simulink model "substation_exp11"  (R2021b)
settings: Solver=VariableStepAuto  StartTime=0.0  StopTime=10  RelTol=1e-3
undefined symbols (not defined in the file): a
libraries: spsThreePhaseBreakerLib x13, spsThreePhaseVIMeasurementLib x10, spsRMSLib x4, spsThreePhaseSeriesRLCLoadLib x4, spsThreePhaseSourceLib x3, spsThreePhaseTransformerTwoWindingsLib x3, spsThreePhaseFaultLib x1, spspowerguiLib x1
settings Model: Creator=SAI KUMAR  LastModifiedBy=SAI KUMAR
settings SolverCC: ZeroCrossAlgorithm=Adaptive
settings DebuggingCC: IgnoredZcDiagnostic=none

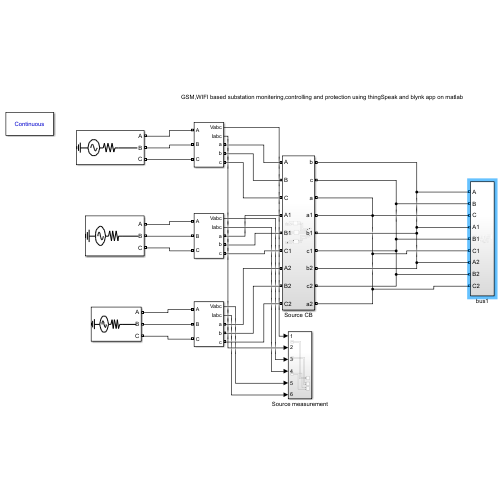
[thumbnail: Simulink's stored preview of the top-level diagram]
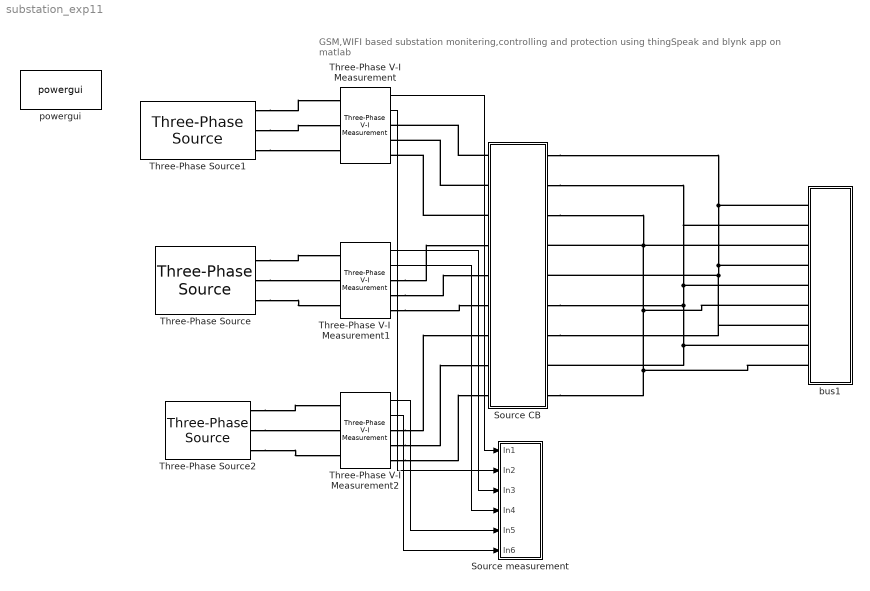
== system substation_exp11 ==
  note: GSM,WIFI based substation monitering,controlling and protection using thingSpeak and blynk app on matlab
  Source CB : Subsystem
  Source measurement : Subsystem
  Three-Phase V-I Measurement : spsThreePhaseVIMeasurementLib/Three-Phase V-I Measurement  VoltageMeasurement=phase-to-ground  SetLabelV=off  LabelV=Vabc  Vpu=off  VpuLL=off  CurrentMeasurement=yes  SetLabelI=off  LabelI=Iabc  Ipu=off  Pbase=100e6  Vbase=500e3  OutputType=Complex  PhasorSimulation=off  PSBequivalent=0
  Three-Phase V-I Measurement1 : spsThreePhaseVIMeasurementLib/Three-Phase V-I Measurement  VoltageMeasurement=phase-to-ground  SetLabelV=off  LabelV=Vabc  Vpu=off  VpuLL=off  CurrentMeasurement=yes  SetLabelI=off  LabelI=Iabc  Ipu=off  Pbase=100e6  Vbase=500e3  OutputType=Complex  PhasorSimulation=off  PSBequivalent=0
  Three-Phase V-I Measurement2 : spsThreePhaseVIMeasurementLib/Three-Phase V-I Measurement  VoltageMeasurement=phase-to-ground  SetLabelV=off  LabelV=Vabc  Vpu=off  VpuLL=off  CurrentMeasurement=yes  SetLabelI=off  LabelI=Iabc  Ipu=off  Pbase=100e6  Vbase=500e3  OutputType=Complex  PhasorSimulation=off  PSBequivalent=0
  Three-Phase Source : spsThreePhaseSourceLib/Three-Phase Source  InternalConnection=Yg  VoltagePhases=off  Voltage=11000  PhaseAngle=0  Voltage_phases=[25e3 25e3 25e3]/sqrt(3)  PhaseAngles_phases=[0 -120 +120]  Frequency=50  NonIdealSource=on  SpecifyImpedance=off  Resistance=0.8929  Inductance=0  ShortCircuitLevel=100e6  BaseVoltage=11000  XRratio=7  BusType=swing  Pref=10e3  Qref=0  Prefabc=[10e3, 10e3, 10e3]  Qrefabc=[0, 0, 0]  Qmin=-inf  Qmax=inf
  Three-Phase Source1 : spsThreePhaseSourceLib/Three-Phase Source  InternalConnection=Yg  VoltagePhases=off  Voltage=11000  PhaseAngle=0  Voltage_phases=[25e3 25e3 25e3]/sqrt(3)  PhaseAngles_phases=[0 -120 +120]  Frequency=50  NonIdealSource=on  SpecifyImpedance=off  Resistance=0.8929  Inductance=0  ShortCircuitLevel=100e6  BaseVoltage=11000  XRratio=7  BusType=swing  Pref=10e3  Qref=0  Prefabc=[10e3, 10e3, 10e3]  Qrefabc=[0, 0, 0]  Qmin=-inf  Qmax=inf
  Three-Phase Source2 : spsThreePhaseSourceLib/Three-Phase Source  InternalConnection=Yg  VoltagePhases=off  Voltage=11000  PhaseAngle=0  Voltage_phases=[25e3 25e3 25e3]/sqrt(3)  PhaseAngles_phases=[0 -120 +120]  Frequency=50  NonIdealSource=on  SpecifyImpedance=off  Resistance=0.8929  Inductance=0  ShortCircuitLevel=100e6  BaseVoltage=11000  XRratio=7  BusType=swing  Pref=10e3  Qref=0  Prefabc=[10e3, 10e3, 10e3]  Qrefabc=[0, 0, 0]  Qmin=-inf  Qmax=inf
  bus1 : Subsystem
  powergui : spspowerguiLib/powergui  Priority=1  SimulationMode=Continuous  SampleTime=50e-6  frequency=60  Iterations=50  frequencyindice=50  Pbase=100e6  ErrMax=1e-4  UnitsV=kV  UnitsW=MW  buscounter=0  FunctionMessages=off  echomessages=off  EnableUseOfTLC=off  CurrentSourceSwitches=off  DisableSnubberDevices=off  DisableRonSwitches=off  DisableVfSwitches=off  DisplayEquations=off  AutomaticDiscreteSolvers=off  SolverType=Tustin/Backward Euler (TBE)  Interpol=off  ExternalGateDelay=off  methode=off  Ts=100  x0status=blocks  SPID=on  SwTol=0  HookPort=off  NonlinearTolerance=1e-4  nMaxIteration=100  ContinueOnMaxIteration=off  RestoreLinks=warning  ResistiveCurrentMeasurement=off  Frange=[0:2:500]  Ylog=off  Xlog=on  ShowGrid=off  save=off  variable=ZData  structure=0  ZoomFFT=off  StartTime=0.0  cycles=1  DisplayStyle=1  fundamental=60  FreqAxis=off  MaxFrequency=1000  frequencyindicesteady=1  RmsSteady=1  display=off
  wires:
  Three-Phase V-I Measurement/1 -> Source measurement/1(In1)
  Three-Phase V-I Measurement/2 -> Source measurement/2(In2)
  Three-Phase V-I Measurement1/1 -> Source measurement/3(In3)
  Three-Phase V-I Measurement1/2 -> Source measurement/4(In4)
  Three-Phase V-I Measurement2/1 -> Source measurement/5(In5)
  Three-Phase V-I Measurement2/2 -> Source measurement/6(In6)
  connections:
  bus1/LConn1 -- Source CB/RConn5 -- Source CB/RConn7 -- bus1/LConn7 -- bus1/LConn4 -- Source CB/RConn1
  Three-Phase Source2/RConn1 -- Three-Phase V-I Measurement2/LConn1
  Three-Phase Source2/RConn2 -- Three-Phase V-I Measurement2/LConn2
  Three-Phase Source2/RConn3 -- Three-Phase V-I Measurement2/LConn3
  Three-Phase Source/RConn1 -- Three-Phase V-I Measurement1/LConn1
  Three-Phase Source/RConn2 -- Three-Phase V-I Measurement1/LConn2
  Three-Phase Source/RConn3 -- Three-Phase V-I Measurement1/LConn3
  Three-Phase Source1/RConn1 -- Three-Phase V-I Measurement/LConn1
  Three-Phase Source1/RConn2 -- Three-Phase V-I Measurement/LConn2
  Three-Phase Source1/RConn3 -- Three-Phase V-I Measurement/LConn3
  bus1/LConn9 -- Source CB/RConn9 -- bus1/LConn6 -- bus1/LConn3 -- Source CB/RConn3 -- Source CB/RConn4
  bus1/LConn5 -- Source CB/RConn2 -- bus1/LConn2 -- Source CB/RConn6 -- Source CB/RConn8 -- bus1/LConn8
  Source CB/LConn1 -- Three-Phase V-I Measurement/RConn1
  Source CB/LConn2 -- Three-Phase V-I Measurement/RConn2
  Source CB/LConn3 -- Three-Phase V-I Measurement/RConn3
  Three-Phase V-I Measurement1/RConn1 -- Source CB/LConn4
  Three-Phase V-I Measurement1/RConn2 -- Source CB/LConn5
  Three-Phase V-I Measurement1/RConn3 -- Source CB/LConn6
  Three-Phase V-I Measurement2/RConn1 -- Source CB/LConn7
  Three-Phase V-I Measurement2/RConn2 -- Source CB/LConn8
  Three-Phase V-I Measurement2/RConn3 -- Source CB/LConn9

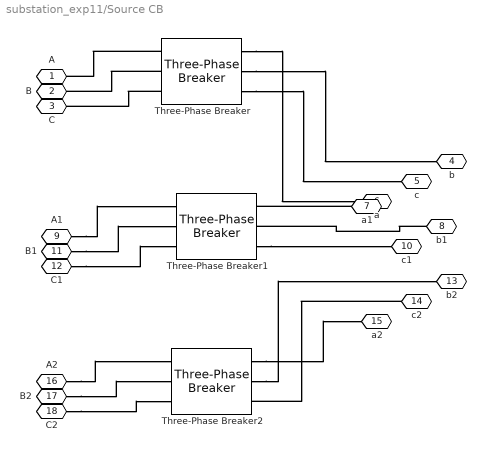
== system substation_exp11/Source CB ==
  Three-Phase Breaker : spsThreePhaseBreakerLib/Three-Phase Breaker  InitialState=closed  SwitchA=on  SwitchB=on  SwitchC=on  SwitchTimes="[1/60  5/60]"  External=off  BreakerResistance=0.01  SnubberResistance=1e6  SnubberCapacitance=inf  Measurements=None
  Three-Phase Breaker1 : spsThreePhaseBreakerLib/Three-Phase Breaker  InitialState=closed  SwitchA=on  SwitchB=on  SwitchC=on  SwitchTimes="[1/60  5/60]"  External=off  BreakerResistance=0.01  SnubberResistance=1e6  SnubberCapacitance=inf  Measurements=None
  Three-Phase Breaker2 : spsThreePhaseBreakerLib/Three-Phase Breaker  InitialState=closed  SwitchA=on  SwitchB=on  SwitchC=on  SwitchTimes="[1/60  5/60]"  External=off  BreakerResistance=0.01  SnubberResistance=1e6  SnubberCapacitance=inf  Measurements=None
  A : PMIOPort  Side=Left
  B : PMIOPort  Port=2  Side=Left
  C : PMIOPort  Port=3  Side=Left
  b : PMIOPort  Port=4  Side=Right
  c : PMIOPort  Port=5  Side=Right
  a : PMIOPort  Port=6  Side=Right
  a1 : PMIOPort  Port=7  Side=Right
  b1 : PMIOPort  Port=8  Side=Right
  A1 : PMIOPort  Port=9  Side=Left
  c1 : PMIOPort  Port=10  Side=Right
  B1 : PMIOPort  Port=11  Side=Left
  C1 : PMIOPort  Port=12  Side=Left
  b2 : PMIOPort  Port=13  Side=Right
  c2 : PMIOPort  Port=14  Side=Right
  a2 : PMIOPort  Port=15  Side=Right
  A2 : PMIOPort  Port=16  Side=Left
  B2 : PMIOPort  Port=17  Side=Left
  C2 : PMIOPort  Port=18  Side=Left
  connections:
  Three-Phase Breaker2/RConn1 -- a2/RConn1
  Three-Phase Breaker2/RConn2 -- b2/RConn1
  A1/RConn1 -- Three-Phase Breaker1/LConn1
  B1/RConn1 -- Three-Phase Breaker1/LConn2
  b1/RConn1 -- Three-Phase Breaker1/RConn2
  C2/RConn1 -- Three-Phase Breaker2/LConn3
  Three-Phase Breaker/RConn1 -- a/RConn1
  c2/RConn1 -- Three-Phase Breaker2/RConn3
  Three-Phase Breaker/RConn3 -- c/RConn1
  Three-Phase Breaker/LConn1 -- A/RConn1
  a1/RConn1 -- Three-Phase Breaker1/RConn1
  B2/RConn1 -- Three-Phase Breaker2/LConn2
  C1/RConn1 -- Three-Phase Breaker1/LConn3
  Three-Phase Breaker/LConn2 -- B/RConn1
  Three-Phase Breaker1/RConn3 -- c1/RConn1
  A2/RConn1 -- Three-Phase Breaker2/LConn1
  Three-Phase Breaker/RConn2 -- b/RConn1
  Three-Phase Breaker/LConn3 -- C/RConn1

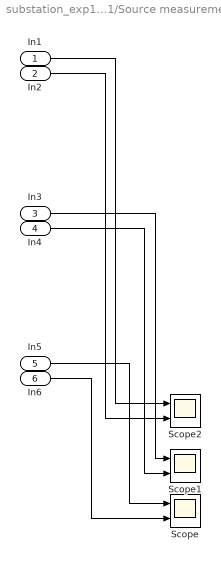
== system substation_exp11/Source measurement ==
  In1 : Inport
  In2 : Inport  Port=2
  In3 : Inport  Port=3
  In4 : Inport  Port=4
  In5 : Inport  Port=5
  In6 : Inport  Port=6
  Scope : Scope  NumInputPorts=2
  Scope1 : Scope  NumInputPorts=2
  Scope2 : Scope  NumInputPorts=2
  wires:
  In5/1 -> Scope/1
  In6/1 -> Scope/2
  In2/1 -> Scope2/2
  In4/1 -> Scope1/2
  In3/1 -> Scope1/1
  In1/1 -> Scope2/1

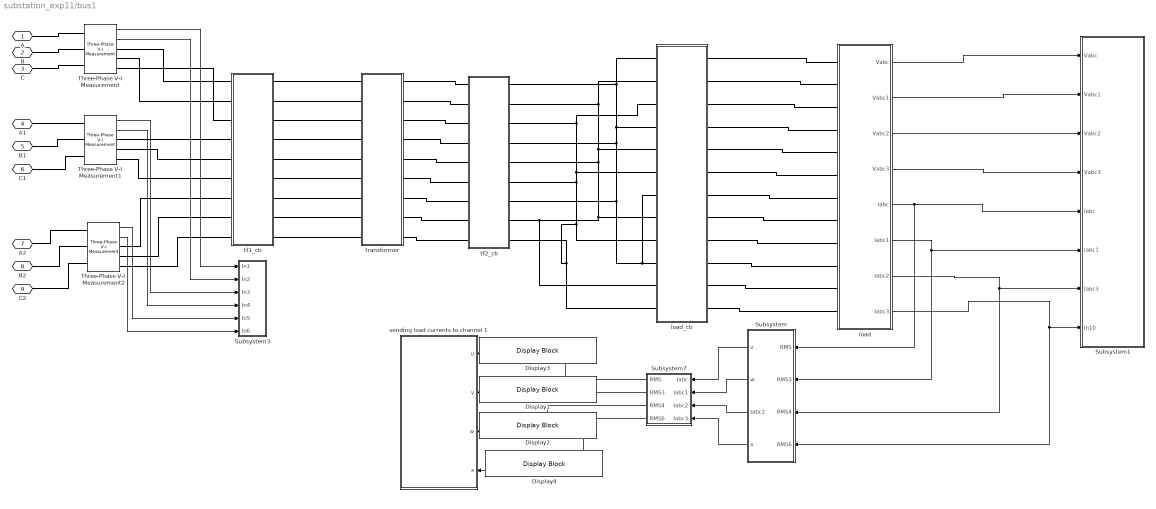
== system substation_exp11/bus1 ==
  Display{1..4} (4 alike) : DisplayBlock  LabelPosition=Hide  Format=short  Transparency=1
  Subsystem : Subsystem
  Subsystem1 : Subsystem
  Subsystem3 : Subsystem
  Subsystem7 : Subsystem
  Three-Phase V-I Measurement : spsThreePhaseVIMeasurementLib/Three-Phase V-I Measurement  VoltageMeasurement=phase-to-ground  SetLabelV=off  LabelV=Vabc  Vpu=off  VpuLL=off  CurrentMeasurement=yes  SetLabelI=off  LabelI=Iabc  Ipu=off  Pbase=100e6  Vbase=500e3  OutputType=Complex  PhasorSimulation=off  PSBequivalent=0
  Three-Phase V-I Measurement1 : spsThreePhaseVIMeasurementLib/Three-Phase V-I Measurement  VoltageMeasurement=phase-to-ground  SetLabelV=off  LabelV=Vabc  Vpu=off  VpuLL=off  CurrentMeasurement=yes  SetLabelI=off  LabelI=Iabc  Ipu=off  Pbase=100e6  Vbase=500e3  OutputType=Complex  PhasorSimulation=off  PSBequivalent=0
  Three-Phase V-I Measurement2 : spsThreePhaseVIMeasurementLib/Three-Phase V-I Measurement  VoltageMeasurement=phase-to-ground  SetLabelV=off  LabelV=Vabc  Vpu=off  VpuLL=off  CurrentMeasurement=yes  SetLabelI=off  LabelI=Iabc  Ipu=off  Pbase=100e6  Vbase=500e3  OutputType=Complex  PhasorSimulation=off  PSBequivalent=0
  load : Subsystem
  load_cb : Subsystem
  sending load currents to channel 1 : MATLAB Function  TreatAsAtomicUnit=on
  tf1_cb : Subsystem
  tf2_cb : Subsystem
  transformer : Subsystem
  A : PMIOPort  Side=Left
  B : PMIOPort  Port=2  Side=Left
  C : PMIOPort  Port=3  Side=Left
  A1 : PMIOPort  Port=4  Side=Left
  B1 : PMIOPort  Port=5  Side=Left
  C1 : PMIOPort  Port=6  Side=Left
  A2 : PMIOPort  Port=7  Side=Left
  B2 : PMIOPort  Port=8  Side=Left
  C2 : PMIOPort  Port=9  Side=Left
  wires:
  Three-Phase V-I Measurement/1 -> Subsystem3/1(In1)
  Three-Phase V-I Measurement/2 -> Subsystem3/2(In2)
  Three-Phase V-I Measurement1/1 -> Subsystem3/3(In3)
  Three-Phase V-I Measurement1/2 -> Subsystem3/4(In4)
  Three-Phase V-I Measurement2/1 -> Subsystem3/5(In5)
  Three-Phase V-I Measurement2/2 -> Subsystem3/6(In6)
  load/6(Iabc1) -> Subsystem1/6(Iabc1), Subsystem/2(RMS3)
  load/8(Iabc3) -> Subsystem/4(RMS6), Subsystem1/8(In10)
  load/1(Vabc) -> Subsystem1/1(Vabc)
  load/2(Vabc1) -> Subsystem1/2(Vabc1)
  load/3(Vabc2) -> Subsystem1/3(Vabc2)
  load/4(Vabc3) -> Subsystem1/4(Vabc3)
  load/5(Iabc) -> Subsystem/1(RMS), Subsystem1/5(Iabc)
  load/7(Iabc2) -> Subsystem/3(RMS4), Subsystem1/7(Iabc3)
  Subsystem/1(v) -> Subsystem7/1(Iabc)
  Subsystem/2(w) -> Subsystem7/2(Iabc1)
  Subsystem/3(Iabc2) -> Subsystem7/3(Iabc2)
  Subsystem/4(x) -> Subsystem7/4(Iabc3)
  Subsystem7/1(RMS) -> sending load currents to channel 1/1(u)
  Subsystem7/2(RMS3) -> sending load currents to channel 1/2(v)
  Subsystem7/3(RMS4) -> sending load currents to channel 1/3(w)
  Subsystem7/4(RMS6) -> sending load currents to channel 1/4(x)
  connections:
  Three-Phase V-I Measurement/LConn1 -- A/RConn1
  Three-Phase V-I Measurement/LConn2 -- B/RConn1
  Three-Phase V-I Measurement/LConn3 -- C/RConn1
  Three-Phase V-I Measurement1/LConn1 -- A1/RConn1
  Three-Phase V-I Measurement1/LConn2 -- B1/RConn1
  Three-Phase V-I Measurement1/LConn3 -- C1/RConn1
  Three-Phase V-I Measurement2/LConn1 -- A2/RConn1
  Three-Phase V-I Measurement2/LConn2 -- B2/RConn1
  Three-Phase V-I Measurement2/LConn3 -- C2/RConn1
  Three-Phase V-I Measurement/RConn1 -- tf1_cb/LConn1
  Three-Phase V-I Measurement/RConn2 -- tf1_cb/LConn2
  Three-Phase V-I Measurement/RConn3 -- tf1_cb/LConn3
  Three-Phase V-I Measurement1/RConn1 -- tf1_cb/LConn4
  Three-Phase V-I Measurement1/RConn2 -- tf1_cb/LConn5
  Three-Phase V-I Measurement1/RConn3 -- tf1_cb/LConn6
  Three-Phase V-I Measurement2/RConn1 -- tf1_cb/LConn7
  Three-Phase V-I Measurement2/RConn2 -- tf1_cb/LConn8
  Three-Phase V-I Measurement2/RConn3 -- tf1_cb/LConn9
  tf2_cb/RConn1 -- tf2_cb/RConn7 -- load_cb/LConn10 -- load_cb/LConn7 -- tf2_cb/RConn4 -- load_cb/LConn4 -- load_cb/LConn1
  tf2_cb/RConn2 -- load_cb/LConn11 -- tf2_cb/RConn8 -- load_cb/LConn8 -- tf2_cb/RConn5 -- load_cb/LConn5 -- load_cb/LConn2
  tf2_cb/RConn3 -- load_cb/LConn12 -- tf2_cb/RConn9 -- load_cb/LConn9 -- tf2_cb/RConn6 -- load_cb/LConn6 -- load_cb/LConn3
  load/LConn1 -- load_cb/RConn1
  load/LConn2 -- load_cb/RConn2
  load_cb/RConn3 -- load/LConn3
  load_cb/RConn4 -- load/LConn4
  load_cb/RConn5 -- load/LConn5
  load_cb/RConn6 -- load/LConn6
  load/LConn7 -- load_cb/RConn7
  load_cb/RConn8 -- load/LConn8
  load_cb/RConn9 -- load/LConn9
  load_cb/RConn10 -- load/LConn10
  load_cb/RConn11 -- load/LConn11
  load_cb/RConn12 -- load/LConn12
  transformer/LConn1 -- tf1_cb/RConn1
  transformer/LConn2 -- tf1_cb/RConn2
  tf2_cb/LConn1 -- transformer/RConn1
  transformer/LConn3 -- tf1_cb/RConn3
  tf2_cb/LConn2 -- transformer/RConn2
  transformer/LConn4 -- tf1_cb/RConn4
  tf2_cb/LConn3 -- transformer/RConn3
  transformer/LConn5 -- tf1_cb/RConn5
  tf2_cb/LConn4 -- transformer/RConn4
  transformer/LConn6 -- tf1_cb/RConn6
  tf2_cb/LConn5 -- transformer/RConn5
  transformer/LConn7 -- tf1_cb/RConn7
  tf2_cb/LConn6 -- transformer/RConn6
  transformer/LConn8 -- tf1_cb/RConn8
  tf2_cb/LConn7 -- transformer/RConn7
  transformer/LConn9 -- tf1_cb/RConn9
  tf2_cb/LConn8 -- transformer/RConn8
  tf2_cb/LConn9 -- transformer/RConn9

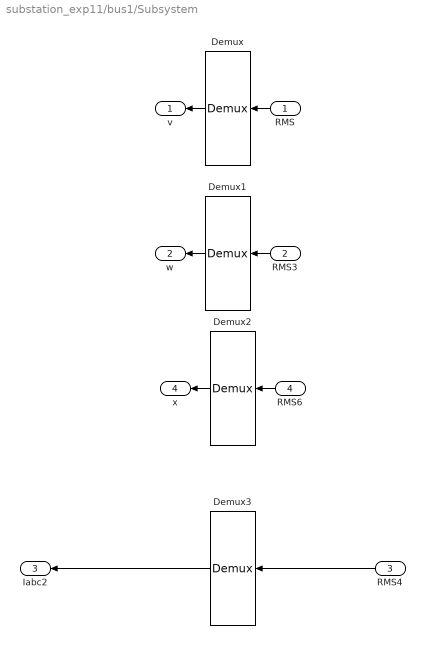
== system substation_exp11/bus1/Subsystem ==
  RMS : Inport
  RMS3 : Inport  Port=2
  RMS4 : Inport  Port=3
  RMS6 : Inport  Port=4
  Demux{,1..3} (4 alike) : Demux  Outputs=3
  v : Outport
  w : Outport  Port=2
  Iabc2 : Outport  Port=3
  x : Outport  Port=4
  wires:
  RMS3/1 -> Demux1/1
  Demux3/2 -> Iabc2/1
  RMS4/1 -> Demux3/1
  Demux1/2 -> w/1
  Demux2/2 -> x/1
  RMS/1 -> Demux/1
  RMS6/1 -> Demux2/1
  Demux/2 -> v/1

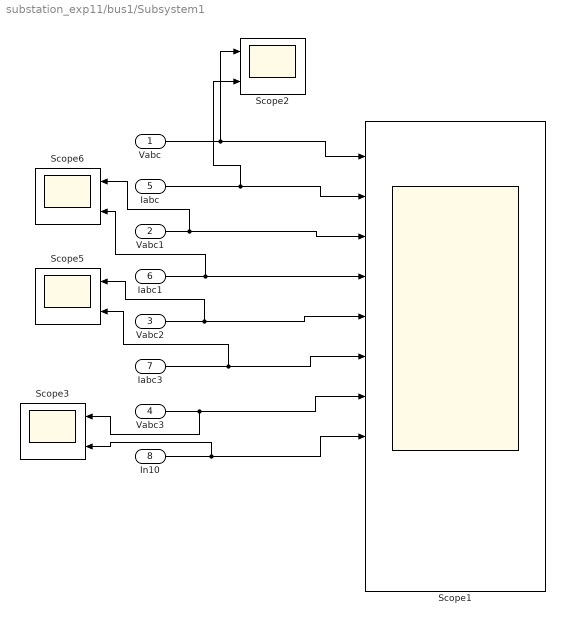
== system substation_exp11/bus1/Subsystem1 ==
  Vabc : Inport
  Vabc1 : Inport  Port=2
  Vabc2 : Inport  Port=3
  Vabc3 : Inport  Port=4
  Iabc : Inport  Port=5
  Iabc1 : Inport  Port=6
  Iabc3 : Inport  Port=7
  In10 : Inport  Port=8
  Scope1 : Scope  NumInputPorts=11
  Scope{2..3,5..6} (4 alike) : Scope  NumInputPorts=2
  wires:
  Iabc3/1 -> Scope5/2, Scope1/6
  Iabc1/1 -> Scope1/4, Scope6/2
  Vabc3/1 -> Scope3/1, Scope1/7
  Vabc2/1 -> Scope5/1, Scope1/5
  Vabc/1 -> Scope2/1, Scope1/1
  Iabc/1 -> Scope2/2, Scope1/2
  Vabc1/1 -> Scope1/3, Scope6/1
  In10/1 -> Scope3/2, Scope1/8

== system substation_exp11/bus1/Subsystem3 ==
  In1 : Inport
  In2 : Inport  Port=2
  In3 : Inport  Port=3
  In4 : Inport  Port=4
  In5 : Inport  Port=5
  In6 : Inport  Port=6
  Scope : Scope  NumInputPorts=2
  Scope3 : Scope  NumInputPorts=2
  Scope4 : Scope  NumInputPorts=2
  wires:
  In4/1 -> Scope3/2
  In1/1 -> Scope/1
  In3/1 -> Scope3/1
  In2/1 -> Scope/2
  In6/1 -> Scope4/2
  In5/1 -> Scope4/1

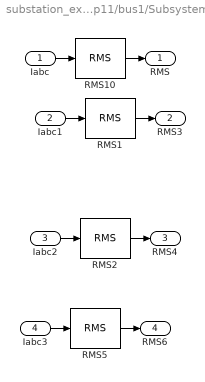
== system substation_exp11/bus1/Subsystem7 ==
  Iabc : Inport
  Iabc1 : Inport  Port=2
  Iabc2 : Inport  Port=3
  Iabc3 : Inport  Port=4
  RMS{1..2,5,10} (4 alike) : spsRMSLib/RMS  TrueRMS=on  Freq=50  RMSInit=0  Ts=a
  RMS : Outport
  RMS3 : Outport  Port=2
  RMS4 : Outport  Port=3
  RMS6 : Outport  Port=4
  wires:
  Iabc1/1 -> RMS1/1
  Iabc2/1 -> RMS2/1
  Iabc3/1 -> RMS5/1
  RMS5/1 -> RMS6/1
  Iabc/1 -> RMS10/1
  RMS2/1 -> RMS4/1
  RMS1/1 -> RMS3/1
  RMS10/1 -> RMS/1

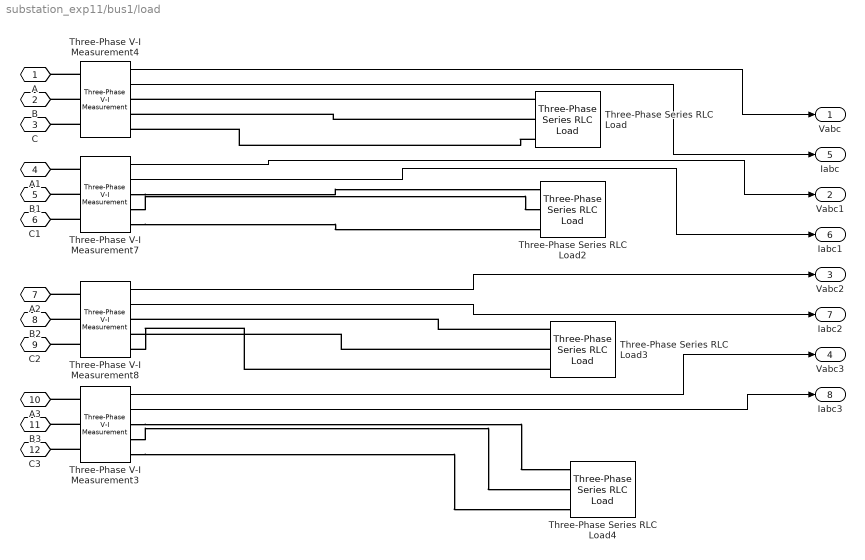
== system substation_exp11/bus1/load ==
  Three-Phase Series RLC Load : spsThreePhaseSeriesRLCLoadLib/Three-Phase Series RLC Load  LConnTagsString=A|B|C  Configuration=Y (grounded)  NominalVoltage=415  Vabc=[1e3 1e3 1e3]  Vabcp=[1e3 1e3 1e3]  NominalFrequency=50  UnbalancedPower=off  ActivePower=1000  InductivePower=0  CapacitivePower=0  Pabc=[10e3 9e3 11e3]  QLabc=[100 90 110]  QCabc=[100 90 110]  Pabcp=[10e3 9e3 11e3]  QLabcp=[100 90 110]  QCabcp=[100 90 110]  Measurements=None  LoadType=constant Z
  Three-Phase Series RLC Load2 : spsThreePhaseSeriesRLCLoadLib/Three-Phase Series RLC Load  LConnTagsString=A|B|C  Configuration=Y (grounded)  NominalVoltage=415  Vabc=[1e3 1e3 1e3]  Vabcp=[1e3 1e3 1e3]  NominalFrequency=50  UnbalancedPower=off  ActivePower=10e3  InductivePower=0  CapacitivePower=0  Pabc=[10e3 9e3 11e3]  QLabc=[100 90 110]  QCabc=[100 90 110]  Pabcp=[10e3 9e3 11e3]  QLabcp=[100 90 110]  QCabcp=[100 90 110]  Measurements=None  LoadType=constant Z
  Three-Phase Series RLC Load3 : spsThreePhaseSeriesRLCLoadLib/Three-Phase Series RLC Load  LConnTagsString=A|B|C  Configuration=Y (grounded)  NominalVoltage=415  Vabc=[1e3 1e3 1e3]  Vabcp=[1e3 1e3 1e3]  NominalFrequency=50  UnbalancedPower=off  ActivePower=10e3  InductivePower=0  CapacitivePower=0  Pabc=[10e3 9e3 11e3]  QLabc=[100 90 110]  QCabc=[100 90 110]  Pabcp=[10e3 9e3 11e3]  QLabcp=[100 90 110]  QCabcp=[100 90 110]  Measurements=None  LoadType=constant Z
  Three-Phase Series RLC Load4 : spsThreePhaseSeriesRLCLoadLib/Three-Phase Series RLC Load  LConnTagsString=A|B|C  Configuration=Y (grounded)  NominalVoltage=415  Vabc=[1e3 1e3 1e3]  Vabcp=[1e3 1e3 1e3]  NominalFrequency=50  UnbalancedPower=off  ActivePower=10e6  InductivePower=0  CapacitivePower=0  Pabc=[10e3 9e3 11e3]  QLabc=[100 90 110]  QCabc=[100 90 110]  Pabcp=[10e3 9e3 11e3]  QLabcp=[100 90 110]  QCabcp=[100 90 110]  Measurements=None  LoadType=constant Z
  Three-Phase V-I Measurement{3..4,7..8} (4 alike) : spsThreePhaseVIMeasurementLib/Three-Phase V-I Measurement  VoltageMeasurement=phase-to-phase  SetLabelV=off  LabelV=Vabc  Vpu=off  VpuLL=off  CurrentMeasurement=yes  SetLabelI=off  LabelI=Iabc  Ipu=off  Pbase=100e6  Vbase=500e3  OutputType=Complex  PhasorSimulation=off  PSBequivalent=0
  A : PMIOPort  Side=Left
  B : PMIOPort  Port=2  Side=Left
  C : PMIOPort  Port=3  Side=Left
  A1 : PMIOPort  Port=4  Side=Left
  B1 : PMIOPort  Port=5  Side=Left
  C1 : PMIOPort  Port=6  Side=Left
  A2 : PMIOPort  Port=7  Side=Left
  B2 : PMIOPort  Port=8  Side=Left
  C2 : PMIOPort  Port=9  Side=Left
  A3 : PMIOPort  Port=10  Side=Left
  B3 : PMIOPort  Port=11  Side=Left
  C3 : PMIOPort  Port=12  Side=Left
  Vabc : Outport
  Vabc1 : Outport  Port=2
  Vabc2 : Outport  Port=3
  Vabc3 : Outport  Port=4
  Iabc : Outport  Port=5
  Iabc1 : Outport  Port=6
  Iabc2 : Outport  Port=7
  Iabc3 : Outport  Port=8
  wires:
  Three-Phase V-I Measurement7/2 -> Iabc1/1
  Three-Phase V-I Measurement4/2 -> Iabc/1
  Three-Phase V-I Measurement8/2 -> Iabc2/1
  Three-Phase V-I Measurement3/1 -> Vabc3/1
  Three-Phase V-I Measurement8/1 -> Vabc2/1
  Three-Phase V-I Measurement4/1 -> Vabc/1
  Three-Phase V-I Measurement7/1 -> Vabc1/1
  Three-Phase V-I Measurement3/2 -> Iabc3/1
  connections:
  Three-Phase V-I Measurement3/RConn2 -- Three-Phase Series RLC Load4/LConn2
  Three-Phase V-I Measurement7/LConn1 -- A1/RConn1
  Three-Phase V-I Measurement7/RConn2 -- Three-Phase Series RLC Load2/LConn2
  Three-Phase V-I Measurement7/RConn3 -- Three-Phase Series RLC Load2/LConn3
  Three-Phase Series RLC Load3/LConn3 -- Three-Phase V-I Measurement8/RConn3
  Three-Phase V-I Measurement8/LConn2 -- B2/RConn1
  Three-Phase Series RLC Load/LConn3 -- Three-Phase V-I Measurement4/RConn3
  Three-Phase Series RLC Load/LConn2 -- Three-Phase V-I Measurement4/RConn2
  Three-Phase Series RLC Load3/LConn2 -- Three-Phase V-I Measurement8/RConn2
  Three-Phase V-I Measurement3/RConn3 -- Three-Phase Series RLC Load4/LConn3
  Three-Phase Series RLC Load3/LConn1 -- Three-Phase V-I Measurement8/RConn1
  Three-Phase V-I Measurement3/RConn1 -- Three-Phase Series RLC Load4/LConn1
  Three-Phase V-I Measurement7/RConn1 -- Three-Phase Series RLC Load2/LConn1
  Three-Phase Series RLC Load/LConn1 -- Three-Phase V-I Measurement4/RConn1
  Three-Phase V-I Measurement7/LConn2 -- B1/RConn1
  Three-Phase V-I Measurement3/LConn1 -- A3/RConn1
  Three-Phase V-I Measurement8/LConn3 -- C2/RConn1
  Three-Phase V-I Measurement8/LConn1 -- A2/RConn1
  Three-Phase V-I Measurement7/LConn3 -- C1/RConn1
  Three-Phase V-I Measurement4/LConn1 -- A/RConn1
  Three-Phase V-I Measurement3/LConn2 -- B3/RConn1
  Three-Phase V-I Measurement4/LConn3 -- C/RConn1
  Three-Phase V-I Measurement4/LConn2 -- B/RConn1
  Three-Phase V-I Measurement3/LConn3 -- C3/RConn1

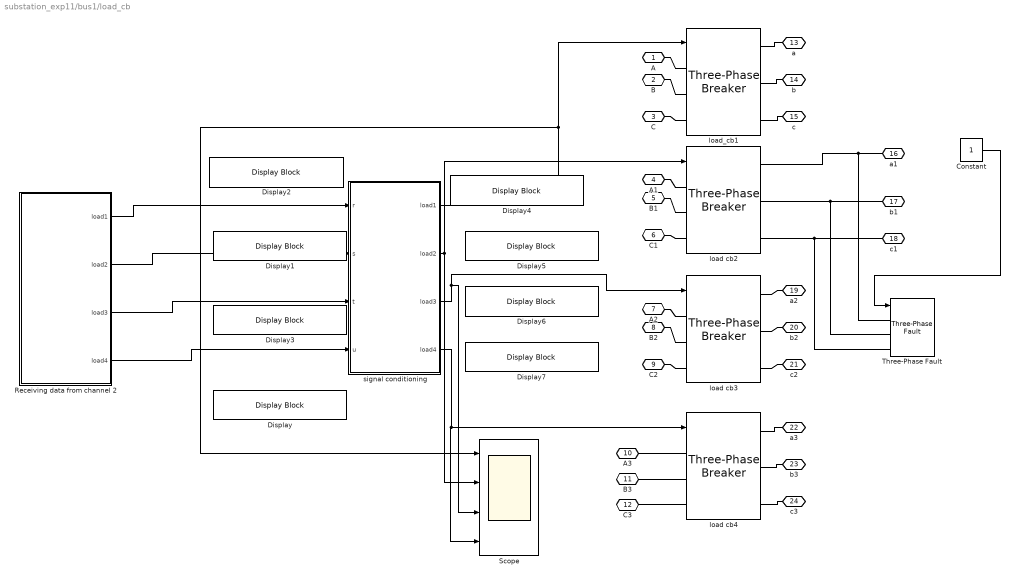
== system substation_exp11/bus1/load_cb ==
  Constant : Constant
  Display{,1..7} (8 alike) : DisplayBlock  LabelPosition=Hide  Format=short  Transparency=1
  Receiving data from channel 2 : MATLAB Function  TreatAsAtomicUnit=on
  Scope : Scope  NumInputPorts=4
  Three-Phase Fault : spsThreePhaseFaultLib/Three-Phase Fault  InitialStates=0  FaultA=on  FaultB=on  FaultC=on  GroundFault=off  SwitchTimes="[1/60  5/60]"  External=on  SwitchStatus=NaN  FaultResistance=0.001  GroundResistance=0.01  SnubberResistance=1e6  SnubberCapacitance=inf  Measurements=None
  load cb2 : spsThreePhaseBreakerLib/Three-Phase Breaker  InitialState=closed  SwitchA=on  SwitchB=on  SwitchC=on  SwitchTimes="[1/60  5/60]"  External=on  BreakerResistance=0.01  SnubberResistance=1e6  SnubberCapacitance=inf  Measurements=None
  load cb3 : spsThreePhaseBreakerLib/Three-Phase Breaker  InitialState=closed  SwitchA=on  SwitchB=on  SwitchC=on  SwitchTimes="[1/60  5/60]"  External=on  BreakerResistance=0.01  SnubberResistance=1e6  SnubberCapacitance=inf  Measurements=None
  load cb4 : spsThreePhaseBreakerLib/Three-Phase Breaker  InitialState=closed  SwitchA=on  SwitchB=on  SwitchC=on  SwitchTimes="[1/60  5/60]"  External=on  BreakerResistance=0.01  SnubberResistance=1e6  SnubberCapacitance=inf  Measurements=None
  load_cb1 : spsThreePhaseBreakerLib/Three-Phase Breaker  InitialState=closed  SwitchA=on  SwitchB=on  SwitchC=on  SwitchTimes="[1/60  5/60]"  External=on  BreakerResistance=0.01  SnubberResistance=1e6  SnubberCapacitance=inf  Measurements=None
  signal conditioning : MATLAB Function  TreatAsAtomicUnit=on
  A : PMIOPort  Side=Left
  B : PMIOPort  Port=2  Side=Left
  C : PMIOPort  Port=3  Side=Left
  A1 : PMIOPort  Port=4  Side=Left
  B1 : PMIOPort  Port=5  Side=Left
  C1 : PMIOPort  Port=6  Side=Left
  A2 : PMIOPort  Port=7  Side=Left
  B2 : PMIOPort  Port=8  Side=Left
  C2 : PMIOPort  Port=9  Side=Left
  A3 : PMIOPort  Port=10  Side=Left
  B3 : PMIOPort  Port=11  Side=Left
  C3 : PMIOPort  Port=12  Side=Left
  a : PMIOPort  Port=13  Side=Right
  b : PMIOPort  Port=14  Side=Right
  c : PMIOPort  Port=15  Side=Right
  a1 : PMIOPort  Port=16  Side=Right
  b1 : PMIOPort  Port=17  Side=Right
  c1 : PMIOPort  Port=18  Side=Right
  a2 : PMIOPort  Port=19  Side=Right
  b2 : PMIOPort  Port=20  Side=Right
  c2 : PMIOPort  Port=21  Side=Right
  a3 : PMIOPort  Port=22  Side=Right
  b3 : PMIOPort  Port=23  Side=Right
  c3 : PMIOPort  Port=24  Side=Right
  wires:
  signal conditioning/1(load1) -> Scope/1, load_cb1/1
  signal conditioning/2(load2) -> load cb2/1, Scope/2
  signal conditioning/3(load3) -> Scope/3, load cb3/1
  signal conditioning/4(load4) -> load cb4/1, Scope/4
  Receiving data from channel 2/1(load1) -> signal conditioning/1(r)
  Receiving data from channel 2/2(load2) -> signal conditioning/2(s)
  Receiving data from channel 2/3(load3) -> signal conditioning/3(t)
  Receiving data from channel 2/4(load4) -> signal conditioning/4(u)
  Constant/1 -> Three-Phase Fault/1
  connections:
  load cb3/LConn1 -- A2/RConn1
  load cb2/LConn1 -- A1/RConn1
  load cb2/RConn1 -- Three-Phase Fault/LConn1 -- a1/RConn1
  load cb3/RConn1 -- a2/RConn1
  load_cb1/RConn1 -- a/RConn1
  load cb4/LConn3 -- C3/RConn1
  load_cb1/LConn2 -- B/RConn1
  load cb4/LConn1 -- A3/RConn1
  load_cb1/LConn1 -- A/RConn1
  load cb2/RConn3 -- Three-Phase Fault/LConn3 -- c1/RConn1
  load cb4/RConn2 -- b3/RConn1
  load cb3/LConn2 -- B2/RConn1
  load cb4/LConn2 -- B3/RConn1
  load cb3/RConn2 -- b2/RConn1
  load cb2/RConn2 -- Three-Phase Fault/LConn2 -- b1/RConn1
  load cb2/LConn2 -- B1/RConn1
  load_cb1/RConn2 -- b/RConn1
  load cb3/LConn3 -- C2/RConn1
  load cb4/RConn1 -- a3/RConn1
  load cb4/RConn3 -- c3/RConn1
  load cb3/RConn3 -- c2/RConn1
  load cb2/LConn3 -- C1/RConn1
  load_cb1/LConn3 -- C/RConn1
  load_cb1/RConn3 -- c/RConn1

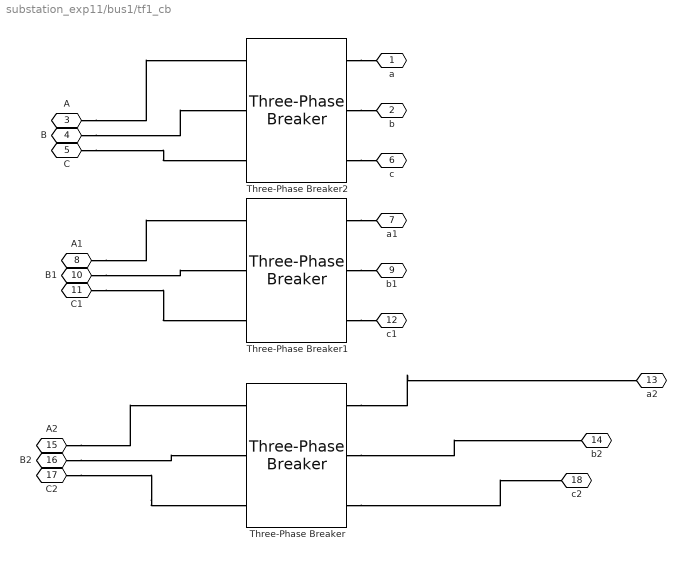
== system substation_exp11/bus1/tf1_cb ==
  Three-Phase Breaker : spsThreePhaseBreakerLib/Three-Phase Breaker  InitialState=closed  SwitchA=on  SwitchB=on  SwitchC=on  SwitchTimes="[1/60  5/60]"  External=off  BreakerResistance=0.01  SnubberResistance=1e6  SnubberCapacitance=inf  Measurements=None
  Three-Phase Breaker1 : spsThreePhaseBreakerLib/Three-Phase Breaker  InitialState=closed  SwitchA=on  SwitchB=on  SwitchC=on  SwitchTimes="[1/60  5/60]"  External=off  BreakerResistance=0.01  SnubberResistance=1e6  SnubberCapacitance=inf  Measurements=None
  Three-Phase Breaker2 : spsThreePhaseBreakerLib/Three-Phase Breaker  InitialState=closed  SwitchA=on  SwitchB=on  SwitchC=on  SwitchTimes="[1/60  5/60]"  External=off  BreakerResistance=0.01  SnubberResistance=1e6  SnubberCapacitance=inf  Measurements=None
  a : PMIOPort  Side=Right
  b : PMIOPort  Port=2  Side=Right
  A : PMIOPort  Port=3  Side=Left
  B : PMIOPort  Port=4  Side=Left
  C : PMIOPort  Port=5  Side=Left
  c : PMIOPort  Port=6  Side=Right
  a1 : PMIOPort  Port=7  Side=Right
  A1 : PMIOPort  Port=8  Side=Left
  b1 : PMIOPort  Port=9  Side=Right
  B1 : PMIOPort  Port=10  Side=Left
  C1 : PMIOPort  Port=11  Side=Left
  c1 : PMIOPort  Port=12  Side=Right
  a2 : PMIOPort  Port=13  Side=Right
  b2 : PMIOPort  Port=14  Side=Right
  A2 : PMIOPort  Port=15  Side=Left
  B2 : PMIOPort  Port=16  Side=Left
  C2 : PMIOPort  Port=17  Side=Left
  c2 : PMIOPort  Port=18  Side=Right
  connections:
  Three-Phase Breaker1/RConn2 -- b1/RConn1
  B1/RConn1 -- Three-Phase Breaker1/LConn2
  Three-Phase Breaker2/RConn1 -- a/RConn1
  Three-Phase Breaker/RConn2 -- b2/RConn1
  Three-Phase Breaker1/RConn3 -- c1/RConn1
  A1/RConn1 -- Three-Phase Breaker1/LConn1
  Three-Phase Breaker2/RConn3 -- c/RConn1
  C1/RConn1 -- Three-Phase Breaker1/LConn3
  Three-Phase Breaker2/RConn2 -- b/RConn1
  Three-Phase Breaker1/RConn1 -- a1/RConn1
  A2/RConn1 -- Three-Phase Breaker/LConn1
  C/RConn1 -- Three-Phase Breaker2/LConn3
  C2/RConn1 -- Three-Phase Breaker/LConn3
  Three-Phase Breaker/RConn1 -- a2/RConn1
  A/RConn1 -- Three-Phase Breaker2/LConn1
  B2/RConn1 -- Three-Phase Breaker/LConn2
  B/RConn1 -- Three-Phase Breaker2/LConn2
  Three-Phase Breaker/RConn3 -- c2/RConn1

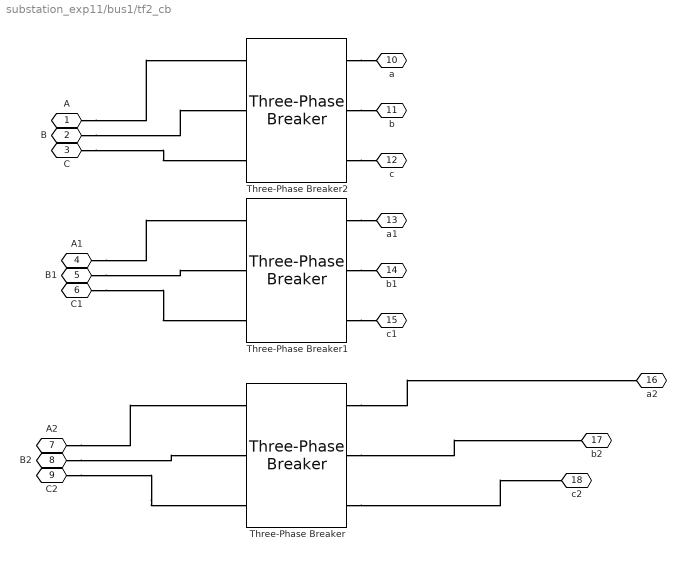
== system substation_exp11/bus1/tf2_cb ==
  Three-Phase Breaker : spsThreePhaseBreakerLib/Three-Phase Breaker  InitialState=closed  SwitchA=on  SwitchB=on  SwitchC=on  SwitchTimes="[1/60  5/60]"  External=off  BreakerResistance=0.01  SnubberResistance=1e6  SnubberCapacitance=inf  Measurements=None
  Three-Phase Breaker1 : spsThreePhaseBreakerLib/Three-Phase Breaker  InitialState=closed  SwitchA=on  SwitchB=on  SwitchC=on  SwitchTimes="[1/60  5/60]"  External=off  BreakerResistance=0.01  SnubberResistance=1e6  SnubberCapacitance=inf  Measurements=None
  Three-Phase Breaker2 : spsThreePhaseBreakerLib/Three-Phase Breaker  InitialState=closed  SwitchA=on  SwitchB=on  SwitchC=on  SwitchTimes="[1/60  5/60]"  External=off  BreakerResistance=0.01  SnubberResistance=1e6  SnubberCapacitance=inf  Measurements=None
  A : PMIOPort  Side=Left
  B : PMIOPort  Port=2  Side=Left
  C : PMIOPort  Port=3  Side=Left
  A1 : PMIOPort  Port=4  Side=Left
  B1 : PMIOPort  Port=5  Side=Left
  C1 : PMIOPort  Port=6  Side=Left
  A2 : PMIOPort  Port=7  Side=Left
  B2 : PMIOPort  Port=8  Side=Left
  C2 : PMIOPort  Port=9  Side=Left
  a : PMIOPort  Port=10  Side=Right
  b : PMIOPort  Port=11  Side=Right
  c : PMIOPort  Port=12  Side=Right
  a1 : PMIOPort  Port=13  Side=Right
  b1 : PMIOPort  Port=14  Side=Right
  c1 : PMIOPort  Port=15  Side=Right
  a2 : PMIOPort  Port=16  Side=Right
  b2 : PMIOPort  Port=17  Side=Right
  c2 : PMIOPort  Port=18  Side=Right
  connections:
  Three-Phase Breaker/RConn3 -- c2/RConn1
  B/RConn1 -- Three-Phase Breaker2/LConn2
  B2/RConn1 -- Three-Phase Breaker/LConn2
  A/RConn1 -- Three-Phase Breaker2/LConn1
  Three-Phase Breaker/RConn1 -- a2/RConn1
  C2/RConn1 -- Three-Phase Breaker/LConn3
  C/RConn1 -- Three-Phase Breaker2/LConn3
  A2/RConn1 -- Three-Phase Breaker/LConn1
  Three-Phase Breaker1/RConn1 -- a1/RConn1
  Three-Phase Breaker2/RConn2 -- b/RConn1
  C1/RConn1 -- Three-Phase Breaker1/LConn3
  Three-Phase Breaker2/RConn3 -- c/RConn1
  A1/RConn1 -- Three-Phase Breaker1/LConn1
  Three-Phase Breaker1/RConn3 -- c1/RConn1
  Three-Phase Breaker/RConn2 -- b2/RConn1
  Three-Phase Breaker2/RConn1 -- a/RConn1
  B1/RConn1 -- Three-Phase Breaker1/LConn2
  Three-Phase Breaker1/RConn2 -- b1/RConn1

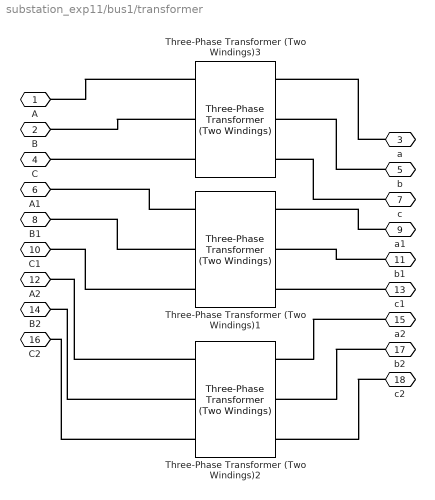
== system substation_exp11/bus1/transformer ==
  Three-Phase Transformer (Two Windings)1 : spsThreePhaseTransformerTwoWindingsLib/Three-Phase Transformer (Two Windings)  Winding1Connection=Yg  Winding2Connection=Yg  CoreType=Three-limb core (core-type)  SetSaturation=off  Hysteresis=off  DataFile='hysteresis'  SetInitialFlux=off  Measurements=None  UNITS=pu  NominalPower=[ 2e6 , 50]  Winding1=[11000 0.002 0.080002]  Winding2=[415 0.002 0.08]  Rm=500  Lm=500  L0=0.5  Saturation=[0 0;0.0024 1.2;1 1.52]  InitialFluxes=[ 0.8 , -0.8 , 0.7 ]  BreakLoop=off  DiscreteSolver=Trapezoidal iterative  DataType=off  TransfoNumber=1
  Three-Phase Transformer (Two Windings)2 : spsThreePhaseTransformerTwoWindingsLib/Three-Phase Transformer (Two Windings)  Winding1Connection=Yg  Winding2Connection=Yg  CoreType=Three-limb core (core-type)  SetSaturation=off  Hysteresis=off  DataFile='hysteresis'  SetInitialFlux=off  Measurements=None  UNITS=pu  NominalPower=[ 2e6 , 50 ]  Winding1=[11000 0.002 0.080002]  Winding2=[415 0.002 0.08]  Rm=500  Lm=500  L0=0.5  Saturation=[0 0;0.0024 1.2;1 1.52]  InitialFluxes=[ 0.8 , -0.8 , 0.7 ]  BreakLoop=off  DiscreteSolver=Trapezoidal iterative  DataType=off  TransfoNumber=1
  Three-Phase Transformer (Two Windings)3 : spsThreePhaseTransformerTwoWindingsLib/Three-Phase Transformer (Two Windings)  Winding1Connection=Yg  Winding2Connection=Yg  CoreType=Three-limb core (core-type)  SetSaturation=off  Hysteresis=off  DataFile='hysteresis'  SetInitialFlux=off  Measurements=None  UNITS=pu  NominalPower=[ 2e6 , 50]  Winding1=[11000 0.002 0.080002]  Winding2=[415 0.002 0.08]  Rm=500  Lm=500  L0=0.5  Saturation=[0 0;0.0024 1.2;1 1.52]  InitialFluxes=[ 0.8 , -0.8 , 0.7 ]  BreakLoop=off  DiscreteSolver=Trapezoidal iterative  DataType=off  TransfoNumber=1
  A : PMIOPort  Side=Left
  B : PMIOPort  Port=2  Side=Left
  a : PMIOPort  Port=3  Side=Right
  C : PMIOPort  Port=4  Side=Left
  b : PMIOPort  Port=5  Side=Right
  A1 : PMIOPort  Port=6  Side=Left
  c : PMIOPort  Port=7  Side=Right
  B1 : PMIOPort  Port=8  Side=Left
  a1 : PMIOPort  Port=9  Side=Right
  C1 : PMIOPort  Port=10  Side=Left
  b1 : PMIOPort  Port=11  Side=Right
  A2 : PMIOPort  Port=12  Side=Left
  c1 : PMIOPort  Port=13  Side=Right
  B2 : PMIOPort  Port=14  Side=Left
  a2 : PMIOPort  Port=15  Side=Right
  C2 : PMIOPort  Port=16  Side=Left
  b2 : PMIOPort  Port=17  Side=Right
  c2 : PMIOPort  Port=18  Side=Right
  connections:
  c1/RConn1 -- Three-Phase Transformer (Two Windings)1/RConn3
  Three-Phase Transformer (Two Windings)3/LConn2 -- B/RConn1
  a2/RConn1 -- Three-Phase Transformer (Two Windings)2/RConn1
  a1/RConn1 -- Three-Phase Transformer (Two Windings)1/RConn1
  c2/RConn1 -- Three-Phase Transformer (Two Windings)2/RConn3
  b2/RConn1 -- Three-Phase Transformer (Two Windings)2/RConn2
  b/RConn1 -- Three-Phase Transformer (Two Windings)3/RConn2
  a/RConn1 -- Three-Phase Transformer (Two Windings)3/RConn1
  Three-Phase Transformer (Two Windings)2/LConn1 -- A2/RConn1
  Three-Phase Transformer (Two Windings)1/LConn1 -- A1/RConn1
  Three-Phase Transformer (Two Windings)1/LConn2 -- B1/RConn1
  c/RConn1 -- Three-Phase Transformer (Two Windings)3/RConn3
  b1/RConn1 -- Three-Phase Transformer (Two Windings)1/RConn2
  Three-Phase Transformer (Two Windings)2/LConn3 -- C2/RConn1
  Three-Phase Transformer (Two Windings)2/LConn2 -- B2/RConn1
  Three-Phase Transformer (Two Windings)3/LConn1 -- A/RConn1
  Three-Phase Transformer (Two Windings)1/LConn3 -- C1/RConn1
  Three-Phase Transformer (Two Windings)3/LConn3 -- C/RConn1

== matlab function substation_exp11/bus1/load_cb/Receiving data from channel 2 ==
  data: load1 output; load2 output; load3 output; load4 output
function [load1,load2,load3,load4] = fcn()
coder.extrinsic("thingSpeakRead");
a=thingSpeakRead(1611357,'Fields',[1,2,3,4],'NumPoints',1,'ReadKey','W1UCA77LJ18VU3XN');
load1=0;
load2=0;
load3=0;
load4=0;
load1=a(1);
load2=a(2);
load3=a(3);
load4=a(4);

== matlab function substation_exp11/bus1/sending load currents to channel 1 ==
  data: u input; v input; w input; x input
function fcn(u, v, w, x)
    
    coder.extrinsic("thingSpeakWrite");
    
    thingSpeakWrite(1561089,"Fields",[1,2,3,4],'Values',[u,v,w,x],'WriteKey','0MT5WK8TP2E0F3ZT');

== matlab function substation_exp11/bus1/load_cb/signal conditioning ==
  data: load1 output; load2 output; load3 output; load4 output; r input; s input; t input; u input
function [load1,load2,load3,load4] = fcn(r,s,t,u)
persistent l;
persistent m;
persistent n;
persistent o;
persistent g;

if(isempty(g))
    l=1;
    m=1;
    n=1;
    o=1;
    g=1;
end


if(isnan(r))
    
    load1=l;
else
    l=r;
    load1=r;
end
 if(isnan(s))
     load2=m;
 else
     m=s;
     load2=s;
 end
 if(isnan(t))
     load3=n;
 else
     n=t;
     load3=t;
 end
 if(isnan(u))
     load4=o;
 else
     o=u;
     load4=u;
 end
end
